simulink model "sim_CTM_2link_arm"  (R2020b)
settings: Solver=FixedStepAuto  StartTime=0.0  StopTime=Tend  FixedStep=Tsim  RelTol=1e-3
values from neighbouring files (symbols this model uses):
  c1 = 0.5    [CTM_2link_arm.m]
  c2 = 0.5    [CTM_2link_arm.m]
  dtheta1_ini = 0    [CTM_2link_arm.m]
  dtheta2_ini = 0    [CTM_2link_arm.m]
  g = 9.8    [CTM_2link_arm.m]
  I1 = M1*l1^2    (= 0.25)    [CTM_2link_arm.m]
  I2 = M2*l2^2    (= 0.25)    [CTM_2link_arm.m]
  kd_1 = 20    [CTM_2link_arm.m]
  kd_2 = 20    [CTM_2link_arm.m]
  ki_1 = 0.1    [CTM_2link_arm.m]
  ki_2 = 0.1    [CTM_2link_arm.m]
  kp_1 = 100    [CTM_2link_arm.m]
  L1 = 1    [CTM_2link_arm.m]
  l1 = 0.5    [CTM_2link_arm.m]
  l2 = 0.5    [CTM_2link_arm.m]
  M1 = 1    [CTM_2link_arm.m]
  M2 = 1    [CTM_2link_arm.m]
  M_0 = [I1+I2+M1*l1^2+M2*L1^2+M2*l2^2 I2+M2*l2^2; I2+M2*l2^2 I2+M2*l2^2]    [CTM_2link_arm.m]
  M_cth2 = [2*M2*L1*l2 M2*L1*l2; M2*L1*l2 0]    [CTM_2link_arm.m]
  theta1_ini = 0    [CTM_2link_arm.m]
  theta2_ini = 0    [CTM_2link_arm.m]
undefined symbols (not defined in the file or in its folder): magnitude
settings Model: Creator=s0612  LastModifiedBy=s0612

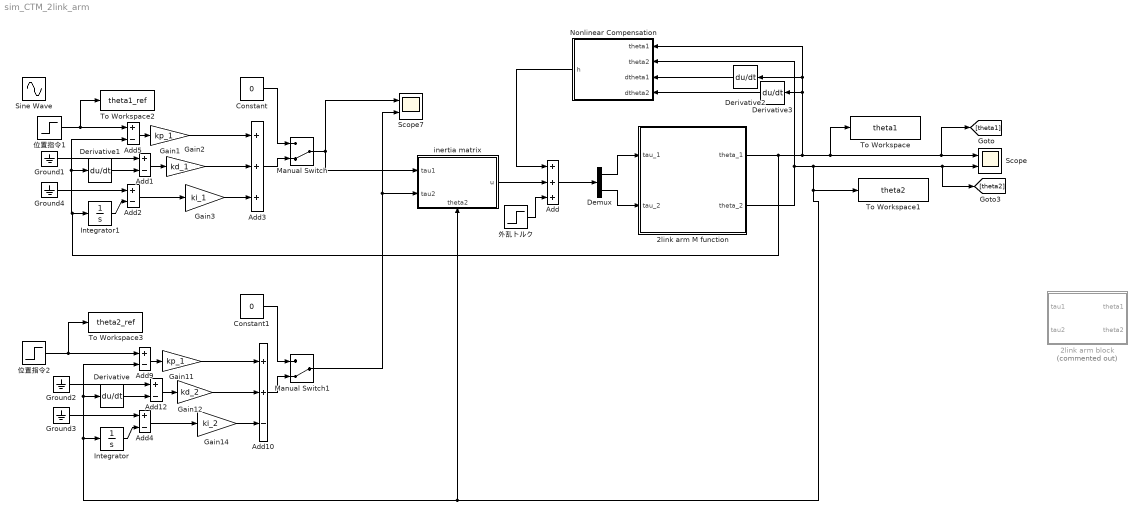
== system sim_CTM_2link_arm ==
  2link arm M function : Subsystem
  2link arm block : Subsystem  Commented=on
  Add : Sum  Inputs=+++
  Add{1..2,4..5,9,12} (6 alike) : Sum  Inputs=+-
  Add10 : Sum  Inputs=++-
  Add3 : Sum  Inputs=+++
  Constant : Constant  Value=0
  Constant1 : Constant  Value=0
  Demux : Demux  Outputs=2
  Derivative{,1..3} (4 alike) : Derivative
  Gain1 : Gain  Gain=kp_1
  Gain11 : Gain  Gain=kp_1
  Gain12 : Gain  Gain=kd_2
  Gain14 : Gain  Gain=ki_2
  Gain2 : Gain  Gain=kd_1
  Gain3 : Gain  Gain=ki_1
  Ground{1..4} (4 alike) : Ground
  Integrator : Integrator
  Integrator1 : Integrator
  Manual Switch : ManualSwitch  CurrentSetting=0
  Manual Switch1 : ManualSwitch  CurrentSetting=0
  Nonlinear Compensation : Subsystem
  Scope : Scope  NumInputPorts=2
  Scope7 : Scope  NumInputPorts=2
  Sine Wave : Sin  Frequency=2*pi*1  SampleTime=0
  To Workspace : ToWorkspace  VariableName=theta1  SaveFormat=Timeseries  SampleTime=-1
  To Workspace1 : ToWorkspace  VariableName=theta2  SaveFormat=Timeseries  SampleTime=-1
  To Workspace2 : ToWorkspace  VariableName=theta1_ref  SaveFormat=Timeseries  SampleTime=-1
  To Workspace3 : ToWorkspace  VariableName=theta2_ref  SaveFormat=Timeseries  SampleTime=-1
  inertia matrix : Subsystem
      settings: PortSchema="{\"entries\":[{\"content\":{\"sides\":[{\"content\":{\"connectorIds\":[\"In1\",\"In2\"]},\"type\":\"ConnectorPlacement.EquallySpacedRectSide\",\"uuid\":\"3e102d75-c9ef-4ca1-acf9-3cfa2777e77b\"},{\"content\":{\"connectorIds\":[\"Out1\"],\"side\":\"RIGHT\"},\"type\":\"ConnectorPlacement.EquallySpacedRectSide\",\"uuid\":\"e376dbc6-2aac-45ab-8f25-30cb7a90e2e9\"},{\"content\":{\"connectorIds\":[],\"side\":\"TOP\"},\"type\":\"ConnectorPlacement.EquallySpacedRectSide\",\"uuid\":\"9022f85b-f286-48be-b339-0cfe4a8b0dbb\"},{\"content\":{\"connectorIds\":[\"In3\"],\"side\":\"BOTTOM\"},\"type\":\"ConnectorPlacement.EquallySpacedRectSide\",\"uuid\":\"2f5ae48a-2d43-4cc2-abb4-5ae82a97453d\"},{\"content\":{\"connectorIds\":[],\"side\":\"HIDDEN\"},\"type\":\"ConnectorPlacement.EquallySpacedRectSide\",\"uuid\":\"e5976d77-d673-4490-92f6-e77791621398\"}]},\"type\":\"ConnectorPlacement.EquallySpacedConnector\",\"uuid\":\"2a9f26fd-748c-421a-9444-f12e0ff06740\"}],\"packageUris\":[\"http://schema.mathworks.com/mf0/Connector/R2020b\"],\"version\":\"1.0\"}"
  位置指令1 : Step  Time=2  After=pi/4  SampleTime=0
  位置指令2 : Step  Time=4  After=pi/2  SampleTime=0
  外乱トルク : Step  Time=7  After=20  SampleTime=0
  wires:
  Manual Switch/1 -> inertia matrix/1(tau1), Scope7/1
  Add3/1 -> Manual Switch/2
  Constant/1 -> Manual Switch/1
  Manual Switch1/1 -> Scope7/2, inertia matrix/2(tau2)
  Constant1/1 -> Manual Switch1/1
  Add10/1 -> Manual Switch1/2
  Add12/1 -> Gain12/1
  Add9/1 -> Gain11/1
  Gain11/1 -> Add10/1
  Gain12/1 -> Add10/2
  Gain3/1 -> Add3/3
  Gain14/1 -> Add10/3
  2link arm M function/2(theta_2) -> Nonlinear Compensation/2(theta2), Derivative/1, Add9/2, Integrator/1, inertia matrix/3(theta2), To Workspace1/1, [theta2], Scope/2
  位置指令2/1 -> To Workspace3/1, Add9/1
  Add4/1 -> Gain14/1
  Ground3/1 -> Add4/1
  Integrator/1 -> Add4/2
  Ground2/1 -> Add12/1
  Derivative/1 -> Add12/2
  2link arm M function/1(theta_1) -> Derivative1/1, Add5/2, Integrator1/1, Nonlinear Compensation/1(theta1), Derivative2/1, Derivative3/1, To Workspace/1, [theta1], Scope/1
  Integrator1/1 -> Add2/2
  Derivative1/1 -> Add1/2
  Ground1/1 -> Add1/1
  Add1/1 -> Gain2/1
  Ground4/1 -> Add2/1
  Add2/1 -> Gain3/1
  Gain2/1 -> Add3/2
  Add5/1 -> Gain1/1
  Gain1/1 -> Add3/1
  位置指令1/1 -> To Workspace2/1, Add5/1
  inertia matrix/1(u) -> Add/2
  Nonlinear Compensation/1(h) -> Add/1
  Add/1 -> Demux/1
  Demux/1 -> 2link arm M function/1(tau_1)
  Demux/2 -> 2link arm M function/2(tau_2)
  Derivative2/1 -> Nonlinear Compensation/3(dtheta1)
  Derivative3/1 -> Nonlinear Compensation/4(dtheta2)
  外乱トルク/1 -> Add/3

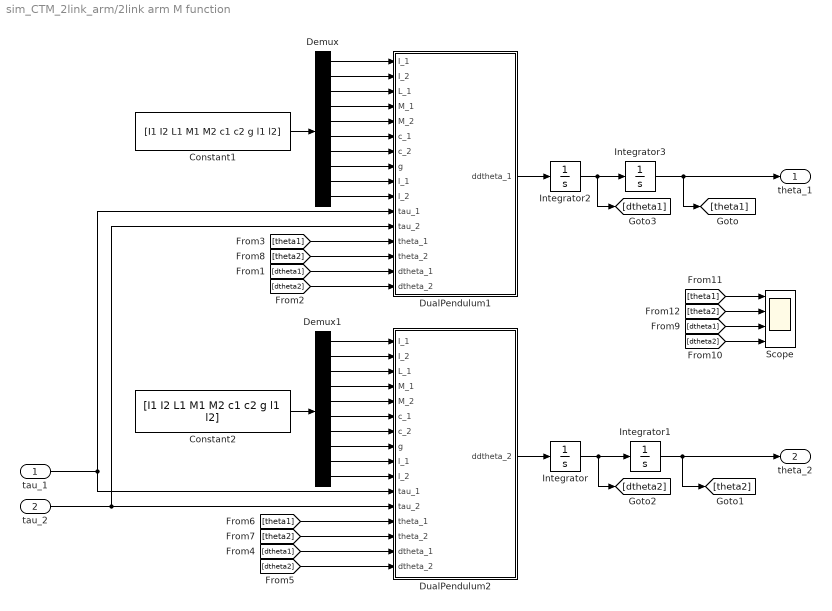
== system sim_CTM_2link_arm/2link arm M function ==
  tau_1 : Inport
  tau_2 : Inport  Port=2
  Constant1 : Constant  Value=[I1 I2 L1 M1 M2 c1 c2 g l1 l2]
  Constant2 : Constant  Value=[I1 I2 L1 M1 M2 c1 c2 g l1 l2]
  Demux : Demux  Outputs=10
  Demux1 : Demux  Outputs=10
  DualPendulum1 : MATLAB Function  TreatAsAtomicUnit=on
  DualPendulum2 : MATLAB Function  TreatAsAtomicUnit=on
  Integrator : Integrator  InitialCondition=dtheta2_ini
  Integrator1 : Integrator  InitialCondition=theta2_ini
  Integrator2 : Integrator  InitialCondition=dtheta1_ini
  Integrator3 : Integrator  InitialCondition=theta1_ini
  Scope : Scope  NumInputPorts=4
  theta_1 : Outport
  theta_2 : Outport  Port=2
  wires:
  Integrator3/1 -> theta_1/1, [theta1]
  Demux/3 -> DualPendulum1/3(L_1)
  Integrator2/1 -> [dtheta1], Integrator3/1
  Demux1/6 -> DualPendulum2/6(c_1)
  [theta1] -> Scope/1
  Demux1/7 -> DualPendulum2/7(c_2)
  Demux1/9 -> DualPendulum2/9(l_1)
  tau_1/1 -> DualPendulum2/11(tau_1), DualPendulum1/11(tau_1)
  [dtheta1] -> Scope/3
  tau_2/1 -> DualPendulum2/12(tau_2), DualPendulum1/12(tau_2)
  Constant1/1 -> Demux/1
  Constant2/1 -> Demux1/1
  [theta2] -> Scope/2
  Demux/7 -> DualPendulum1/7(c_2)
  Demux1/2 -> DualPendulum2/2(I_2)
  Integrator/1 -> Integrator1/1, [dtheta2]
  [dtheta1] -> DualPendulum1/15(dtheta_1)
  Integrator1/1 -> theta_2/1, [theta2]
  Demux1/5 -> DualPendulum2/5(M_2)
  Demux1/8 -> DualPendulum2/8(g)
  DualPendulum2/1(ddtheta_2) -> Integrator/1
  Demux/1 -> DualPendulum1/1(I_1)
  Demux/5 -> DualPendulum1/5(M_2)
  [dtheta2] -> Scope/4
  [dtheta2] -> DualPendulum2/16(dtheta_2)
  Demux1/10 -> DualPendulum2/10(l_2)
  Demux/10 -> DualPendulum1/10(l_2)
  [dtheta2] -> DualPendulum1/16(dtheta_2)
  Demux1/4 -> DualPendulum2/4(M_1)
  Demux1/3 -> DualPendulum2/3(L_1)
  [theta2] -> DualPendulum2/14(theta_2)
  [theta1] -> DualPendulum2/13(theta_1)
  [dtheta1] -> DualPendulum2/15(dtheta_1)
  Demux1/1 -> DualPendulum2/1(I_1)
  Demux/8 -> DualPendulum1/8(g)
  [theta2] -> DualPendulum1/14(theta_2)
  [theta1] -> DualPendulum1/13(theta_1)
  DualPendulum1/1(ddtheta_1) -> Integrator2/1
  Demux/6 -> DualPendulum1/6(c_1)
  Demux/2 -> DualPendulum1/2(I_2)
  Demux/4 -> DualPendulum1/4(M_1)
  Demux/9 -> DualPendulum1/9(l_1)

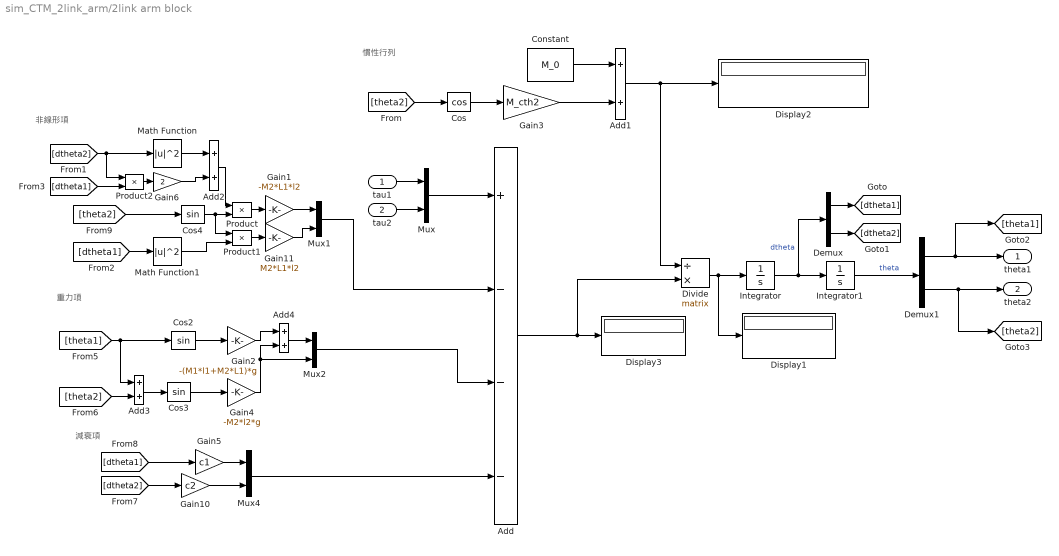
== system sim_CTM_2link_arm/2link arm block ==
  note: 慣性行列
  note: 減衰項
  note: 重力項
  note: 非線形項
  tau1 : Inport
  tau2 : Inport  Port=2
  Add : Sum  Inputs=+---
  Add{1..4} (4 alike) : Sum
  Constant : Constant  Value=M_0
  Cos : Trigonometry  Operator=cos
  Cos2 : Trigonometry
  Cos3 : Trigonometry
  Cos4 : Trigonometry
  Demux : Demux  Outputs=2
  Demux1 : Demux  Outputs=2
  Display1 : Display
  Display2 : Display
  Display3 : Display
  Divide : Product  Inputs=/*  Multiplication=Matrix(*)
  Gain1 : Gain  Gain=-M2*L1*l2
  Gain10 : Gain  Gain=c2
  Gain11 : Gain  Gain=M2*L1*l2
  Gain2 : Gain  Gain=-(M1*l1+M2*L1)*g
  Gain3 : Gain  Gain=M_cth2
  Gain4 : Gain  Gain=-M2*l2*g
  Gain5 : Gain  Gain=c1
  Gain6 : Gain  Gain=2
  Integrator : Integrator  InitialCondition=[dtheta1_ini; dtheta2_ini]
  Integrator1 : Integrator  InitialCondition=[theta1_ini; theta2_ini]
  Math Function : Math  Operator=magnitude^2  SaturateOnIntegerOverflow=on
  Math Function1 : Math  Operator=magnitude^2  SaturateOnIntegerOverflow=on
  Mux{,1..2,4} (4 alike) : Mux  Inputs=2
  Product : Product
  Product1 : Product
  Product2 : Product
  theta1 : Outport
  theta2 : Outport  Port=2
  wires:
  Integrator/1 -> Integrator1/1, Demux/1  "dtheta"
  Mux/1 -> Add/1
  Demux/1 -> [dtheta1]
  Demux/2 -> [dtheta2]
  Integrator1/1 -> Demux1/1  "theta"
  Demux1/2 -> [theta2], theta2/1
  Constant/1 -> Add1/1
  tau1/1 -> Mux/1
  tau2/1 -> Mux/2
  Mux1/1 -> Add/2
  [dtheta1] -> Math Function1/1
  Mux2/1 -> Add/3
  [theta1] -> Add3/1, Cos2/1
  Cos2/1 -> Gain2/1
  Mux4/1 -> Add/4
  [dtheta2] -> Gain10/1
  [dtheta1] -> Gain5/1
  Gain3/1 -> Add1/2
  Divide/1 -> Integrator/1, Display1/1
  Add/1 -> Display3/1, Divide/2
  Demux1/1 -> theta1/1, [theta1]
  [theta2] -> Cos/1
  Add3/1 -> Cos3/1
  Gain2/1 -> Add4/1
  Cos3/1 -> Gain4/1
  Gain4/1 -> Mux2/2, Add4/2
  [theta2] -> Cos4/1
  Cos4/1 -> Product1/1, Product/2
  [dtheta2] -> Product2/1, Math Function/1
  Product/1 -> Gain1/1
  Gain1/1 -> Mux1/1
  Gain5/1 -> Mux4/1
  Gain10/1 -> Mux4/2
  Cos/1 -> Gain3/1
  Gain11/1 -> Mux1/2
  Product1/1 -> Gain11/1
  Math Function1/1 -> Product1/2
  Add1/1 -> Divide/1, Display2/1
  [theta2] -> Add3/2
  Add4/1 -> Mux2/1
  [dtheta1] -> Product2/2
  Product2/1 -> Gain6/1
  Math Function/1 -> Add2/1
  Gain6/1 -> Add2/2
  Add2/1 -> Product/1

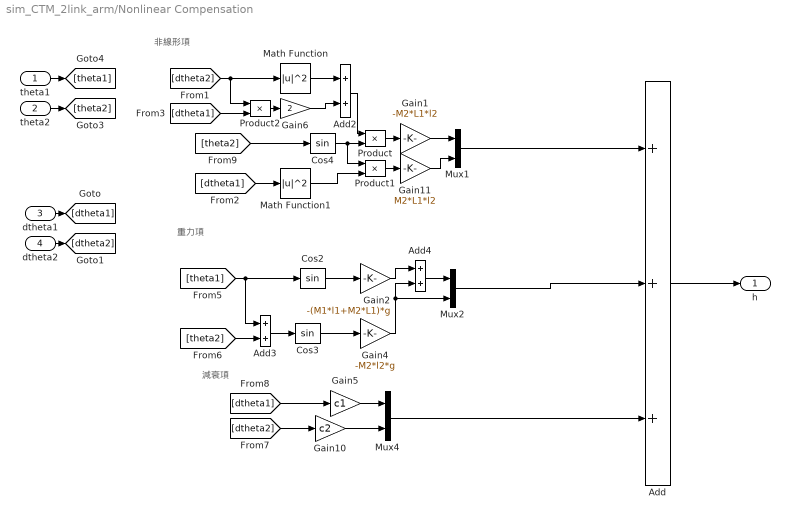
== system sim_CTM_2link_arm/Nonlinear Compensation ==
  note: 減衰項
  note: 重力項
  note: 非線形項
  theta1 : Inport
  theta2 : Inport  Port=2
  dtheta1 : Inport  Port=3
  dtheta2 : Inport  Port=4
  Add : Sum  Inputs=+++
  Add2 : Sum
  Add3 : Sum
  Add4 : Sum
  Cos2 : Trigonometry
  Cos3 : Trigonometry
  Cos4 : Trigonometry
  Gain1 : Gain  Gain=-M2*L1*l2
  Gain10 : Gain  Gain=c2
  Gain11 : Gain  Gain=M2*L1*l2
  Gain2 : Gain  Gain=-(M1*l1+M2*L1)*g
  Gain4 : Gain  Gain=-M2*l2*g
  Gain5 : Gain  Gain=c1
  Gain6 : Gain  Gain=2
  Math Function : Math  Operator=magnitude^2  SaturateOnIntegerOverflow=on
  Math Function1 : Math  Operator=magnitude^2  SaturateOnIntegerOverflow=on
  Mux1 : Mux  Inputs=2
  Mux2 : Mux  Inputs=2
  Mux4 : Mux  Inputs=2
  Product : Product
  Product1 : Product
  Product2 : Product
  h : Outport
  wires:
  Mux1/1 -> Add/1
  [dtheta1] -> Math Function1/1
  Mux2/1 -> Add/2
  [theta1] -> Add3/1, Cos2/1
  Cos2/1 -> Gain2/1
  Mux4/1 -> Add/3
  [dtheta2] -> Gain10/1
  [dtheta1] -> Gain5/1
  Add/1 -> h/1
  Add3/1 -> Cos3/1
  Gain2/1 -> Add4/1
  Cos3/1 -> Gain4/1
  Gain4/1 -> Mux2/2, Add4/2
  [theta2] -> Cos4/1
  Cos4/1 -> Product1/1, Product/2
  [dtheta2] -> Product2/1, Math Function/1
  Product/1 -> Gain1/1
  Gain1/1 -> Mux1/1
  Gain5/1 -> Mux4/1
  Gain10/1 -> Mux4/2
  Gain11/1 -> Mux1/2
  Product1/1 -> Gain11/1
  Math Function1/1 -> Product1/2
  [theta2] -> Add3/2
  Add4/1 -> Mux2/1
  [dtheta1] -> Product2/2
  Product2/1 -> Gain6/1
  Math Function/1 -> Add2/1
  Gain6/1 -> Add2/2
  Add2/1 -> Product/1
  theta1/1 -> [theta1]
  theta2/1 -> [theta2]
  dtheta2/1 -> [dtheta2]
  dtheta1/1 -> [dtheta1]

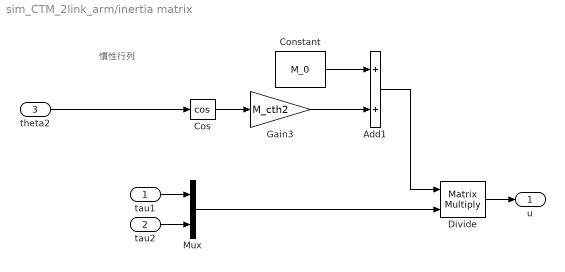
== system sim_CTM_2link_arm/inertia matrix ==
  note: 慣性行列
  tau1 : Inport
  tau2 : Inport  Port=2
  theta2 : Inport  Port=3
  Add1 : Sum
  Constant : Constant  Value=M_0
  Cos : Trigonometry  Operator=cos
  Divide : Product  Inputs=**  Multiplication=Matrix(*)
  Gain3 : Gain  Gain=M_cth2
  Mux : Mux  Inputs=2
  u : Outport
  wires:
  Constant/1 -> Add1/1
  tau1/1 -> Mux/1
  tau2/1 -> Mux/2
  Gain3/1 -> Add1/2
  Divide/1 -> u/1
  Mux/1 -> Divide/2
  theta2/1 -> Cos/1
  Cos/1 -> Gain3/1
  Add1/1 -> Divide/1

== matlab function sim_CTM_2link_arm/2link arm M function/DualPendulum2 ==
  data: I_1 input; ddtheta_2 output; I_2 input; L_1 input; M_1 input; M_2 input; c_1 input; c_2 input; g input; l_1 input; l_2 input; tau_1 input; tau_2 input; theta_1 input; theta_2 input; dtheta_1 input; dtheta_2 input
function ddtheta_2 = DualPendulum2(I_1,I_2,L_1,M_1,M_2,c_1,c_2,g,l_1,l_2,tau_1,tau_2,theta_1,theta_2,dtheta_1,dtheta_2)
%#codegen

%    This function was generated by the Symbolic Math Toolbox version 8.7.
%    25-Nov-2022 09:23:53

t2 = cos(theta_1);
t3 = sin(theta_1);
t4 = theta_1+theta_2;
t5 = L_1.^2;
t6 = L_1.^3;
t7 = M_2.^2;
t8 = dtheta_1.^2;
t9 = dtheta_2.^2;
t10 = l_1.^2;
t11 = l_2.^2;
t12 = l_2.^3;
t13 = t2.^2;
t14 = t2.^3;
t15 = t3.^2;
t16 = t3.^3;
t17 = cos(t4);
t18 = sin(t4);
t19 = t17.^2;
t20 = t17.^3;
t21 = t18.^2;
t22 = t18.^3;
et1 = -I_1.*tau_2+I_2.*tau_1-I_2.*tau_2-I_2.*c_1.*dtheta_1+I_1.*c_2.*dtheta_2+I_2.*c_2.*dtheta_2-M_2.*t5.*t13.*tau_2-M_2.*t5.*t15.*tau_2-M_1.*t10.*t13.*tau_2-M_1.*t10.*t15.*tau_2+M_2.*t11.*t19.*tau_1-M_2.*t11.*t19.*tau_2+M_2.*t11.*t21.*tau_1-M_2.*t11.*t21.*tau_2+I_2.*L_1.*M_2.*g.*t3+I_2.*M_1.*g.*l_1.*t3-I_1.*M_2.*g.*l_2.*t18+M_2.*c_2.*dtheta_2.*t5.*t13+M_2.*c_2.*dtheta_2.*t5.*t15+M_1.*c_2.*dtheta_2.*t10.*t13+M_1.*c_2.*dtheta_2.*t10.*t15-M_2.*c_1.*dtheta_1.*t11.*t19-M_2.*c_1.*dtheta_1.*t11.*t21+M_2.*c_2.*dtheta_2.*t11.*t19+M_2.*c_2.*dtheta_2.*t11.*t21-g.*l_2.*t5.*t7.*t13.*t18+l_2.*t6.*t7.*t8.*t14.*t18-l_2.*t6.*t7.*t8.*t16.*t17+L_1.*M_2.*l_2.*t2.*t17.*tau_1-L_1.*M_2.*l_2.*t2.*t17.*tau_2.*2.0+L_1.*M_2.*l_2.*t3.*t18.*tau_1;
et2 = L_1.*M_2.*l_2.*t3.*t18.*tau_2.*-2.0+L_1.*g.*t3.*t7.*t11.*t19-L_1.*t3.*t7.*t8.*t12.*t20+L_1.*t2.*t7.*t8.*t12.*t22-L_1.*t3.*t7.*t9.*t12.*t20+L_1.*t2.*t7.*t9.*t12.*t22+I_1.*L_1.*M_2.*l_2.*t2.*t8.*t18-I_1.*L_1.*M_2.*l_2.*t3.*t8.*t17+I_2.*L_1.*M_2.*l_2.*t2.*t8.*t18-I_2.*L_1.*M_2.*l_2.*t3.*t8.*t17+I_2.*L_1.*M_2.*l_2.*t2.*t9.*t18-I_2.*L_1.*M_2.*l_2.*t3.*t9.*t17-L_1.*M_2.*c_1.*dtheta_1.*l_2.*t2.*t17-L_1.*M_2.*c_1.*dtheta_1.*l_2.*t3.*t18+L_1.*M_2.*c_2.*dtheta_2.*l_2.*t2.*t17.*2.0+L_1.*M_2.*c_2.*dtheta_2.*l_2.*t3.*t18.*2.0+M_1.*M_2.*g.*l_1.*t3.*t11.*t19+M_1.*M_2.*g.*l_1.*t3.*t11.*t21-M_1.*M_2.*g.*l_2.*t10.*t13.*t18-M_1.*M_2.*g.*l_2.*t10.*t15.*t18-L_1.*dtheta_1.*dtheta_2.*t3.*t7.*t12.*t20.*2.0+L_1.*dtheta_1.*dtheta_2.*t2.*t7.*t12.*t22.*2.0;
et3 = -L_1.*g.*t2.*t7.*t11.*t17.*t18+L_1.*t2.*t7.*t8.*t12.*t18.*t19+L_1.*t2.*t7.*t9.*t12.*t18.*t19-L_1.*t3.*t7.*t8.*t12.*t17.*t21-L_1.*t3.*t7.*t9.*t12.*t17.*t21+g.*l_2.*t2.*t3.*t5.*t7.*t17-l_2.*t3.*t6.*t7.*t8.*t13.*t17+l_2.*t2.*t6.*t7.*t8.*t15.*t18-t2.*t3.*t5.*t7.*t8.*t11.*t19.*2.0-t2.*t3.*t5.*t7.*t9.*t11.*t19+t2.*t3.*t5.*t7.*t8.*t11.*t21.*2.0+t2.*t3.*t5.*t7.*t9.*t11.*t21+t5.*t7.*t8.*t11.*t13.*t17.*t18.*2.0+t5.*t7.*t9.*t11.*t13.*t17.*t18-t5.*t7.*t8.*t11.*t15.*t17.*t18.*2.0-t5.*t7.*t9.*t11.*t15.*t17.*t18+I_2.*L_1.*M_2.*dtheta_1.*dtheta_2.*l_2.*t2.*t18.*2.0-I_2.*L_1.*M_2.*dtheta_1.*dtheta_2.*l_2.*t3.*t17.*2.0+L_1.*M_1.*M_2.*g.*l_1.*l_2.*t15.*t18+L_1.*M_1.*M_2.*l_2.*t8.*t10.*t14.*t18-L_1.*M_1.*M_2.*l_2.*t8.*t10.*t16.*t17;
et4 = L_1.*dtheta_1.*dtheta_2.*t2.*t7.*t12.*t18.*t19.*2.0-L_1.*dtheta_1.*dtheta_2.*t3.*t7.*t12.*t17.*t21.*2.0-dtheta_1.*dtheta_2.*t2.*t3.*t5.*t7.*t11.*t19.*2.0+dtheta_1.*dtheta_2.*t2.*t3.*t5.*t7.*t11.*t21.*2.0+dtheta_1.*dtheta_2.*t5.*t7.*t11.*t13.*t17.*t18.*2.0-dtheta_1.*dtheta_2.*t5.*t7.*t11.*t15.*t17.*t18.*2.0+L_1.*M_1.*M_2.*g.*l_1.*l_2.*t2.*t3.*t17-L_1.*M_1.*M_2.*l_2.*t3.*t8.*t10.*t13.*t17+L_1.*M_1.*M_2.*l_2.*t2.*t8.*t10.*t15.*t18;
ddtheta_2 = -(et1+et2+et3+et4)./(I_1.*I_2+I_2.*M_2.*t5.*t13+I_2.*M_2.*t5.*t15+I_2.*M_1.*t10.*t13+I_2.*M_1.*t10.*t15+I_1.*M_2.*t11.*t19+I_1.*M_2.*t11.*t21+t5.*t7.*t11.*t13.*t21+t5.*t7.*t11.*t15.*t19+M_1.*M_2.*t10.*t11.*t13.*t19+M_1.*M_2.*t10.*t11.*t13.*t21+M_1.*M_2.*t10.*t11.*t15.*t19+M_1.*M_2.*t10.*t11.*t15.*t21-t2.*t3.*t5.*t7.*t11.*t17.*t18.*2.0);

== matlab function sim_CTM_2link_arm/2link arm M function/DualPendulum1 ==
  data: I_1 input; ddtheta_1 output; I_2 input; L_1 input; M_1 input; M_2 input; c_1 input; c_2 input; g input; l_1 input; l_2 input; tau_1 input; tau_2 input; theta_1 input; theta_2 input; dtheta_1 input; dtheta_2 input
function ddtheta_1 = DualPendulum1(I_1,I_2,L_1,M_1,M_2,c_1,c_2,g,l_1,l_2,tau_1,tau_2,theta_1,theta_2,dtheta_1,dtheta_2)
%#codegen

%    This function was generated by the Symbolic Math Toolbox version 8.7.
%    25-Nov-2022 09:23:53

t2 = cos(theta_1);
t3 = sin(theta_1);
t4 = theta_1+theta_2;
t5 = L_1.^2;
t6 = M_2.^2;
t7 = dtheta_1.^2;
t8 = dtheta_2.^2;
t9 = l_1.^2;
t10 = l_2.^2;
t11 = l_2.^3;
t12 = t2.^2;
t13 = t3.^2;
t14 = cos(t4);
t15 = sin(t4);
t16 = t14.^2;
t17 = t14.^3;
t18 = t15.^2;
t19 = t15.^3;
et1 = I_2.*tau_1-I_2.*tau_2-I_2.*c_1.*dtheta_1+I_2.*c_2.*dtheta_2+M_2.*t10.*t16.*tau_1-M_2.*t10.*t16.*tau_2+M_2.*t10.*t18.*tau_1-M_2.*t10.*t18.*tau_2+I_2.*L_1.*M_2.*g.*t3+I_2.*M_1.*g.*l_1.*t3-M_2.*c_1.*dtheta_1.*t10.*t16-M_2.*c_1.*dtheta_1.*t10.*t18+M_2.*c_2.*dtheta_2.*t10.*t16+M_2.*c_2.*dtheta_2.*t10.*t18-L_1.*M_2.*l_2.*t2.*t14.*tau_2-L_1.*M_2.*l_2.*t3.*t15.*tau_2+L_1.*g.*t3.*t6.*t10.*t16-L_1.*t3.*t6.*t7.*t11.*t17+L_1.*t2.*t6.*t7.*t11.*t19-L_1.*t3.*t6.*t8.*t11.*t17+L_1.*t2.*t6.*t8.*t11.*t19+I_2.*L_1.*M_2.*l_2.*t2.*t7.*t15-I_2.*L_1.*M_2.*l_2.*t3.*t7.*t14+I_2.*L_1.*M_2.*l_2.*t2.*t8.*t15-I_2.*L_1.*M_2.*l_2.*t3.*t8.*t14+L_1.*M_2.*c_2.*dtheta_2.*l_2.*t2.*t14+L_1.*M_2.*c_2.*dtheta_2.*l_2.*t3.*t15+M_1.*M_2.*g.*l_1.*t3.*t10.*t16;
et2 = M_1.*M_2.*g.*l_1.*t3.*t10.*t18-L_1.*dtheta_1.*dtheta_2.*t3.*t6.*t11.*t17.*2.0+L_1.*dtheta_1.*dtheta_2.*t2.*t6.*t11.*t19.*2.0-L_1.*g.*t2.*t6.*t10.*t14.*t15+L_1.*t2.*t6.*t7.*t11.*t15.*t16+L_1.*t2.*t6.*t8.*t11.*t15.*t16-L_1.*t3.*t6.*t7.*t11.*t14.*t18-L_1.*t3.*t6.*t8.*t11.*t14.*t18-t2.*t3.*t5.*t6.*t7.*t10.*t16+t2.*t3.*t5.*t6.*t7.*t10.*t18+t5.*t6.*t7.*t10.*t12.*t14.*t15-t5.*t6.*t7.*t10.*t13.*t14.*t15+I_2.*L_1.*M_2.*dtheta_1.*dtheta_2.*l_2.*t2.*t15.*2.0-I_2.*L_1.*M_2.*dtheta_1.*dtheta_2.*l_2.*t3.*t14.*2.0+L_1.*dtheta_1.*dtheta_2.*t2.*t6.*t11.*t15.*t16.*2.0-L_1.*dtheta_1.*dtheta_2.*t3.*t6.*t11.*t14.*t18.*2.0;
ddtheta_1 = (et1+et2)./(I_1.*I_2+I_2.*M_2.*t5.*t12+I_2.*M_2.*t5.*t13+I_2.*M_1.*t9.*t12+I_2.*M_1.*t9.*t13+I_1.*M_2.*t10.*t16+I_1.*M_2.*t10.*t18+t5.*t6.*t10.*t13.*t16+t5.*t6.*t10.*t12.*t18+M_1.*M_2.*t9.*t10.*t12.*t16+M_1.*M_2.*t9.*t10.*t13.*t16+M_1.*M_2.*t9.*t10.*t12.*t18+M_1.*M_2.*t9.*t10.*t13.*t18-t2.*t3.*t5.*t6.*t10.*t14.*t15.*2.0);
